simulink model "TallerSenales2"  (R2016a)
settings: Solver=VariableStepAuto  StartTime=0.0  StopTime=10.0  RelTol=1e-3
settings Model: Creator=USUARIO  LastModifiedBy=sebas

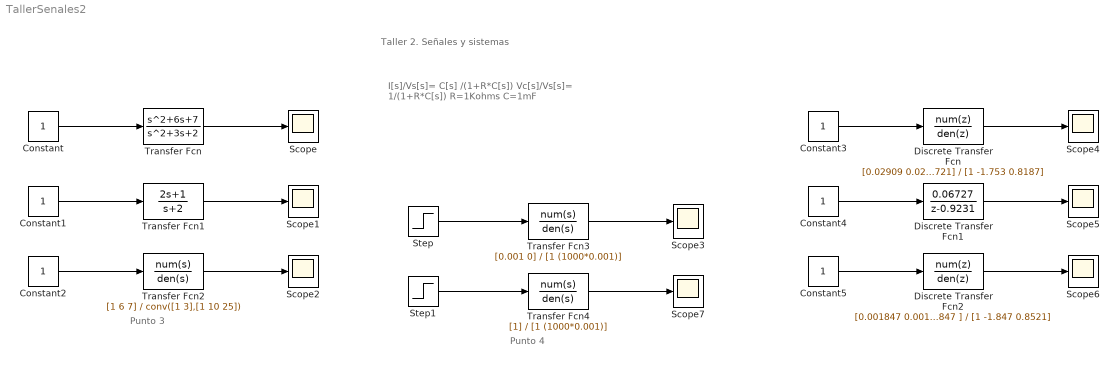
== system TallerSenales2 ==
  note: I[s]/Vs[s]= C[s] /(1+R*C[s])
      |
      | Vc[s]/Vs[s]= 1/(1+R*C[s])
      |
      | R=1Kohms
      | C=1mF
  note: Taller 2. Señales y sistemas
  note: Punto 3
  note: Punto 4
  Constant{,1..5} (6 alike) : Constant
  Discrete Transfer Fcn : DiscreteTransferFcn  Numerator=[0.02909 0.02721]  Denominator=[1 -1.753 0.8187]  SampleTime=0.1
  Discrete Transfer Fcn1 : DiscreteTransferFcn  Numerator=[0.06727]  Denominator=[1 -0.9231]  SampleTime=0.1
  Discrete Transfer Fcn2 : DiscreteTransferFcn  Numerator=[0.001847 0.001847 ]  Denominator=[1 -1.847 0.8521]  SampleTime=0.1
  Scope{,1..7} (8 alike) : Scope
  Step : Step  Time=0  SampleTime=0
  Step1 : Step  Time=0  SampleTime=0
  Transfer Fcn : TransferFcn  Numerator=[1 6 7]  Denominator=[1 3 2]
  Transfer Fcn1 : TransferFcn  Numerator=[2 1]  Denominator=[1 2]
  Transfer Fcn2 : TransferFcn  Numerator=[1 6 7]  Denominator=conv([1 3],[1 10 25])
  Transfer Fcn3 : TransferFcn  Numerator=[0.001 0]  Denominator=[1 (1000*0.001)]
  Transfer Fcn4 : TransferFcn  Denominator=[1 (1000*0.001)]
  wires:
  Transfer Fcn/1 -> Scope/1
  Constant/1 -> Transfer Fcn/1
  Transfer Fcn1/1 -> Scope1/1
  Constant1/1 -> Transfer Fcn1/1
  Transfer Fcn2/1 -> Scope2/1
  Constant2/1 -> Transfer Fcn2/1
  Transfer Fcn3/1 -> Scope3/1
  Step/1 -> Transfer Fcn3/1
  Discrete Transfer Fcn/1 -> Scope4/1
  Constant3/1 -> Discrete Transfer Fcn/1
  Discrete Transfer Fcn1/1 -> Scope5/1
  Constant4/1 -> Discrete Transfer Fcn1/1
  Discrete Transfer Fcn2/1 -> Scope6/1
  Constant5/1 -> Discrete Transfer Fcn2/1
  Transfer Fcn4/1 -> Scope7/1
  Step1/1 -> Transfer Fcn4/1
